simulink model "Ex2_7"  (R2016a)
settings: Solver=VariableStepAuto  StartTime=0.0  StopTime=5  RelTol=1e-3
settings Model: Creator=mende  LastModifiedBy=mende

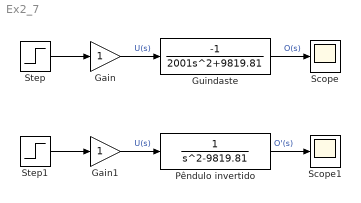
== system Ex2_7 ==
  Gain : Gain
  Gain1 : Gain
  Guindaste : TransferFcn  Numerator=[-1]  Denominator=[2001 0 9819.81]
  Pêndulo invertido : TransferFcn  Denominator=[1 0 -9819.81]
  Scope : Scope
  Scope1 : Scope
  Step : Step  SampleTime=0
  Step1 : Step  SampleTime=0
  wires:
  Step/1 -> Gain/1
  Gain/1 -> Guindaste/1  "U(s)"
  Guindaste/1 -> Scope/1  "O(s)"
  Step1/1 -> Gain1/1
  Gain1/1 -> Pêndulo invertido/1  "U(s)"
  Pêndulo invertido/1 -> Scope1/1  "O'(s)"
